simulink model "PI_Controller"  (R2020a)
settings: Solver=ode15s  StartTime=0.0  StopTime=30  MaxStep=0.1  RelTol=1e-3
settings Model: DataDictionary=Ques_3_Parameters.sldd  Creator=DELL  LastModifiedBy=DELL
settings DataIOCC: SaveOutput=off  SaveTime=off

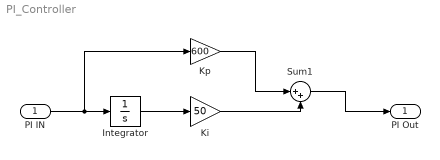
== system PI_Controller ==
  PI IN : Inport  OutDataTypeStr=double  PortDimensions=1  SampleTime=0
  Integrator : Integrator
  Ki : Gain  Gain=50
  Kp : Gain  Gain=600
  Sum1 : Sum  Inputs=|++
  PI Out : Outport  OutDataTypeStr=double  PortDimensions=1  SampleTime=0
  wires:
  Ki/1 -> Sum1/2
  PI IN/1 -> Kp/1, Integrator/1
  Kp/1 -> Sum1/1
  Sum1/1 -> PI Out/1
  Integrator/1 -> Ki/1
